simulink model "oya2"  (R2015a)
settings: Solver=ode45  StartTime=0.0  StopTime=20.0  RelTol=1e-3
settings Model: Creator=yusuke  LastModifiedBy=yusuke

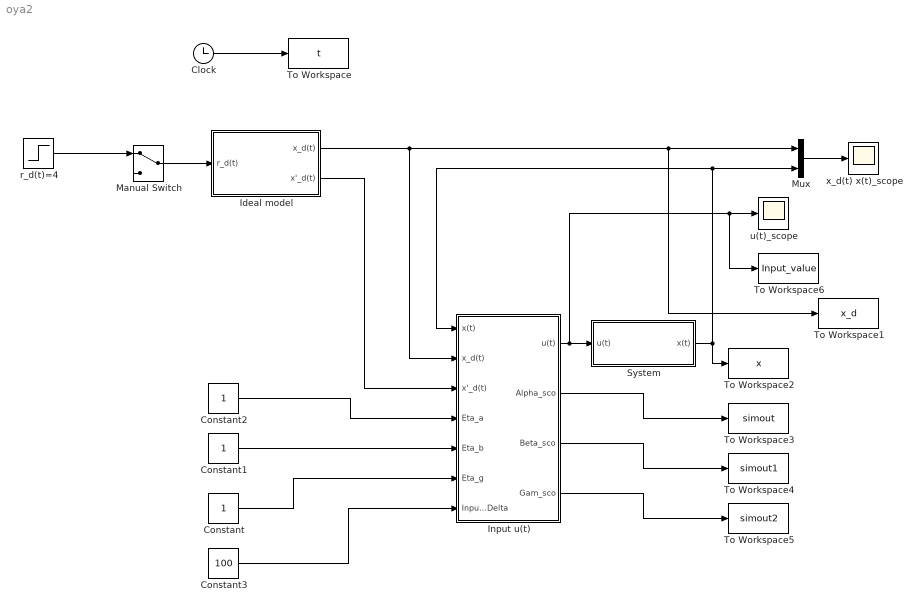
== system oya2 ==
  Clock : Clock
  Constant : Constant
  Constant1 : Constant
  Constant2 : Constant
  Constant3 : Constant  Value=100
  Ideal model : Subsystem
  Input u(t) : Subsystem
  Manual Switch : ManualSwitch
  Mux : Mux  Inputs=2
  System : Subsystem
  To Workspace : ToWorkspace  VariableName=t  SaveFormat=Timeseries  SampleTime=-1
  To Workspace1 : ToWorkspace  VariableName=x_d  SaveFormat=Timeseries  SampleTime=-1
  To Workspace2 : ToWorkspace  VariableName=x  SaveFormat=Timeseries  SampleTime=-1
  To Workspace3 : ToWorkspace  VariableName=simout  SaveFormat=Timeseries  SampleTime=-1
  To Workspace4 : ToWorkspace  VariableName=simout1  SaveFormat=Timeseries  SampleTime=-1
  To Workspace5 : ToWorkspace  VariableName=simout2  SaveFormat=Timeseries  SampleTime=-1
  To Workspace6 : ToWorkspace  VariableName=Input_value  SaveFormat=Timeseries  SampleTime=-1
  r_d(t)=4 : Step  Time=0  After=4  SampleTime=0
  u(t)_scope : Scope
      settings: YMin=-500  YMax=10500
  x_d(t) x(t)_scope : Scope
  wires:
  Manual Switch/1 -> Ideal model/1(r_d(t))
  Clock/1 -> To Workspace/1
  Mux/1 -> x_d(t) x(t)_scope/1
  Ideal model/1(x_d(t)) -> Input u(t)/2(x_d(t)), Mux/1, To Workspace1/1
  System/1(x(t)) -> Input u(t)/1(x(t)), Mux/2, To Workspace2/1
  Input u(t)/1(u(t)) -> To Workspace6/1, u(t)_scope/1, System/1(u(t))
  Input u(t)/2(Alpha_sco) -> To Workspace3/1
  Input u(t)/3(Beta_sco) -> To Workspace4/1
  Input u(t)/4(Gam_sco) -> To Workspace5/1
  Ideal model/2(x'_d(t)) -> Input u(t)/3(x'_d(t))
  Constant3/1 -> Input u(t)/7(Input_Delta)
  Constant/1 -> Input u(t)/6(Eta_g)
  Constant1/1 -> Input u(t)/5(Eta_b)
  Constant2/1 -> Input u(t)/4(Eta_a)
  r_d(t)=4/1 -> Manual Switch/1

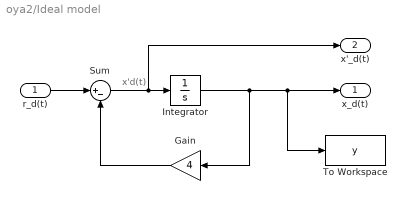
== system oya2/Ideal model ==
  note: x'd(t)
  r_d(t) : Inport
  Gain : Gain  Gain=4
  Integrator : Integrator
  Sum : Sum  Inputs=|+-
  To Workspace : ToWorkspace  VariableName=y  SaveFormat=Timeseries  SampleTime=-1
  x_d(t) : Outport
  x'_d(t) : Outport  Port=2
  wires:
  Integrator/1 -> Gain/1, To Workspace/1, x_d(t)/1
  r_d(t)/1 -> Sum/1
  Sum/1 -> Integrator/1, x'_d(t)/1
  Gain/1 -> Sum/2

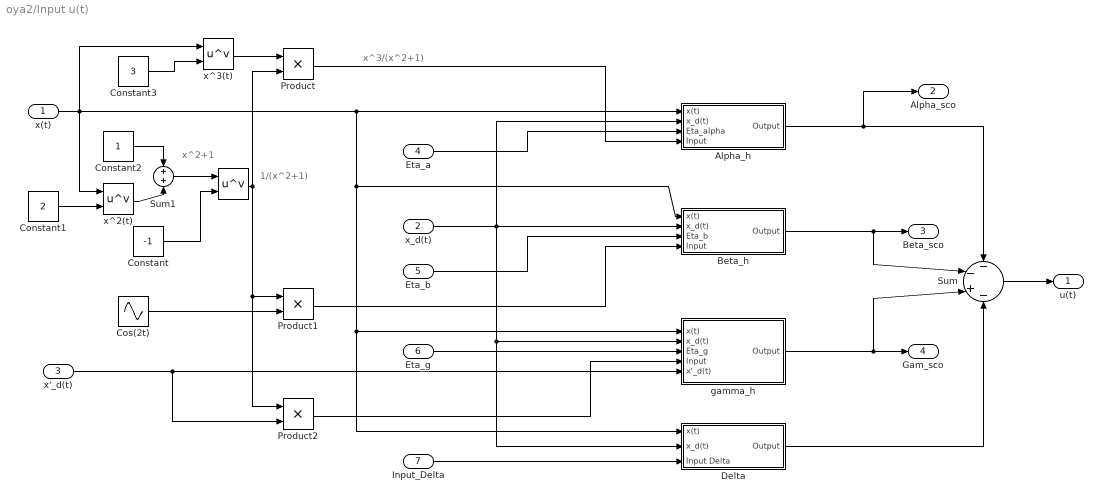
== system oya2/Input u(t) ==
  note: x^3/(x^2+1)
  note: x^2+1
  note: 1/(x^2+1)
  x(t) : Inport
  x_d(t) : Inport  Port=2
  x'_d(t) : Inport  Port=3
  Eta_a : Inport  Port=4
  Eta_b : Inport  Port=5
  Eta_g : Inport  Port=6
  Input_Delta : Inport  Port=7
  " " : Math  Operator=pow  SaturateOnIntegerOverflow=on
  " x^2(t)" : Math  Operator=pow  SaturateOnIntegerOverflow=on
  Alpha_h : Subsystem
  Beta_h : Subsystem
  Constant : Constant  Value=-1
  Constant1 : Constant  Value=2
  Constant2 : Constant
  Constant3 : Constant  Value=3
  Cos(2t) : Sin  Frequency=2  SampleTime=0
  Delta : Subsystem
  Product : Product
  Product1 : Product
  Product2 : Product
  Sum : Sum  Inputs=--+-
  Sum1 : Sum  Inputs=+|+
  gamma_h : Subsystem
  x^3(t) : Math  Operator=pow  SaturateOnIntegerOverflow=on
  u(t) : Outport
  Alpha_sco : Outport  Port=2
  Beta_sco : Outport  Port=3
  Gam_sco : Outport  Port=4
  wires:
  Sum/1 -> u(t)/1
  Delta/1("Output ") -> Sum/4
  gamma_h/1(Output) -> Gam_sco/1, Sum/3
  Beta_h/1(Output) -> Beta_sco/1, Sum/2
  Alpha_h/1(Output) -> Alpha_sco/1, Sum/1
  x(t)/1 -> Alpha_h/1(x(t)), Delta/1(x(t)), gamma_h/1(x(t)), Beta_h/1(x(t)), x^3(t)/1, " x^2(t)"/1
  x_d(t)/1 -> gamma_h/2(x_d(t)), Delta/2(x_d(t)), Beta_h/2(x_d(t)), Alpha_h/2(x_d(t))
  Eta_a/1 -> Alpha_h/3(Eta_alpha)
  Eta_b/1 -> Beta_h/3(Eta_b)
  Eta_g/1 -> gamma_h/3(Eta_g)
  x'_d(t)/1 -> Product2/2, gamma_h/5(x'_d(t))
  Input_Delta/1 -> Delta/3(Input Delta)
  Constant/1 -> " "/2
  Constant1/1 -> " x^2(t)"/2
  Constant2/1 -> Sum1/1
  " x^2(t)"/1 -> Sum1/2
  Sum1/1 -> " "/1
  Constant3/1 -> x^3(t)/2
  x^3(t)/1 -> Product/1
  " "/1 -> Product/2, Product2/1, Product1/1
  Product/1 -> Alpha_h/4(Input)
  Cos(2t)/1 -> Product1/2
  Product1/1 -> Beta_h/4(Input)
  Product2/1 -> gamma_h/4(Input)

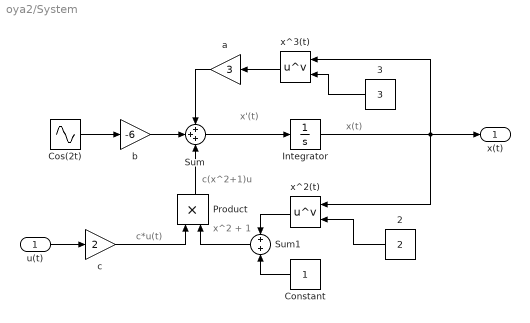
== system oya2/System ==
  note: c(x^2+1)u
  note: c*u(t)
  note: x^2 + 1
  note: x'(t)
  note: x(t)
  u(t) : Inport
  2 : Constant  Value=2
  3 : Constant  Value=3
  Constant : Constant
  Cos(2t) : Sin  Frequency=2  Phase=pi/2  SampleTime=0
  Integrator : Integrator
  Product : Product
  Sum : Sum  Inputs=+++
  Sum1 : Sum  Inputs=+|+
  a : Gain  Gain=3
  b : Gain  Gain=-6
  c : Gain  Gain=2
  x^2(t) : Math  Operator=pow  SaturateOnIntegerOverflow=on
  x^3(t) : Math  Operator=pow  SaturateOnIntegerOverflow=on
  x(t) : Outport
  wires:
  u(t)/1 -> c/1
  Integrator/1 -> x^2(t)/1, x^3(t)/1, x(t)/1
  2/1 -> x^2(t)/2
  Cos(2t)/1 -> b/1
  3/1 -> x^3(t)/2
  Sum/1 -> Integrator/1
  c/1 -> Product/1
  b/1 -> Sum/2
  Product/1 -> Sum/3
  x^2(t)/1 -> Sum1/1
  Constant/1 -> Sum1/2
  Sum1/1 -> Product/2
  x^3(t)/1 -> a/1
  a/1 -> Sum/1

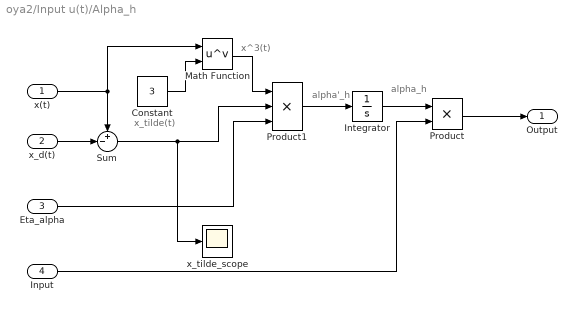
== system oya2/Input u(t)/Alpha_h ==
  note: alpha'_h
  note: alpha_h
  note: x^3(t)
  note: x_tilde(t)
  x(t) : Inport
  x_d(t) : Inport  Port=2
  Eta_alpha : Inport  Port=3
  Input : Inport  Port=4
  Constant : Constant  Value=3
  Integrator : Integrator
  Math Function : Math  Operator=pow  SaturateOnIntegerOverflow=on
  Product : Product
  Product1 : Product  Inputs=3
  Sum : Sum  Inputs=+-|
  x_tilde_scope : Scope
      settings: YMin=-1  YMax=1  SaveName=ScopeData2
  Output : Outport
  wires:
  Product/1 -> Output/1
  Input/1 -> Product/2
  Integrator/1 -> Product/1
  Product1/1 -> Integrator/1
  Eta_alpha/1 -> Product1/3
  x_d(t)/1 -> Sum/2
  Sum/1 -> x_tilde_scope/1, Product1/2
  x(t)/1 -> Sum/1, Math Function/1
  Constant/1 -> Math Function/2
  Math Function/1 -> Product1/1

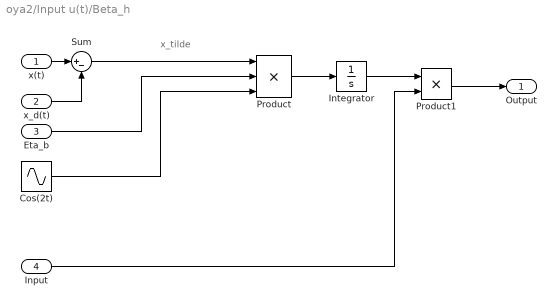
== system oya2/Input u(t)/Beta_h ==
  note: x_tilde
  x(t) : Inport
  x_d(t) : Inport  Port=2
  Eta_b : Inport  Port=3
  Input : Inport  Port=4
  Cos(2t) : Sin  Frequency=2  Phase=pi/2  SampleTime=0
  Integrator : Integrator
  Product : Product  Inputs=3
  Product1 : Product
  Sum : Sum  Inputs=|+-
  Output : Outport
  wires:
  x(t)/1 -> Sum/1
  x_d(t)/1 -> Sum/2
  Sum/1 -> Product/1
  Eta_b/1 -> Product/2
  Cos(2t)/1 -> Product/3
  Product/1 -> Integrator/1
  Integrator/1 -> Product1/1
  Product1/1 -> Output/1
  Input/1 -> Product1/2

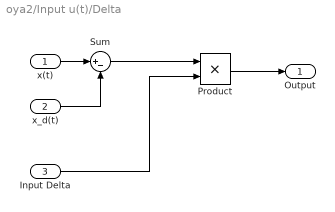
== system oya2/Input u(t)/Delta ==
  x(t) : Inport
  x_d(t) : Inport  Port=2
  Input Delta : Inport  Port=3
  Product : Product
  Sum : Sum  Inputs=|+-
  "Output " : Outport
  wires:
  x(t)/1 -> Sum/1
  x_d(t)/1 -> Sum/2
  Sum/1 -> Product/1
  Product/1 -> "Output "/1
  Input Delta/1 -> Product/2

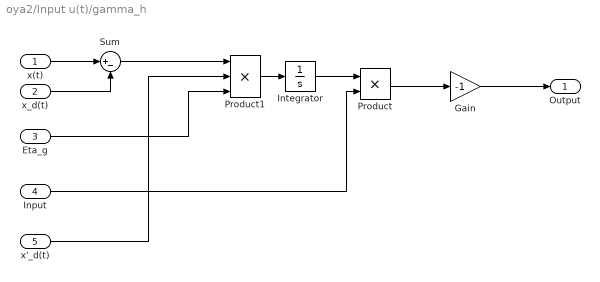
== system oya2/Input u(t)/gamma_h ==
  x(t) : Inport
  x_d(t) : Inport  Port=2
  Eta_g : Inport  Port=3
  Input : Inport  Port=4
  x'_d(t) : Inport  Port=5
  Gain : Gain  Gain=-1
  Integrator : Integrator
  Product : Product
  Product1 : Product  Inputs=3
  Sum : Sum  Inputs=|+-
  Output : Outport
  wires:
  x(t)/1 -> Sum/1
  x_d(t)/1 -> Sum/2
  Integrator/1 -> Product/1
  Input/1 -> Product/2
  Product1/1 -> Integrator/1
  Sum/1 -> Product1/1
  Eta_g/1 -> Product1/3
  Product/1 -> Gain/1
  Gain/1 -> Output/1
  x'_d(t)/1 -> Product1/2
